simulink model "simple_wind_turbine_pmsg"  (Simulink 10.0)
settings: Solver=ode23tb  StartTime=0.0  StopTime=2  MaxStep=0.04  RelTol=1e-3  EnableMultiTasking=on
libraries: powerlib x5, simulink x1, powerlib_extras x1, re_lib x1
Description:
  | This model is developed to encourage the learner/student to develop a
  | Variable Speed Wind Turbine with PMSG. I considered basic parameters
  | in Matlab Blocks with little modification based on the output/load.
  | User can vary and simulate any parameter to study the response of
  | the system.
  | User can add a rectifier and a battery for battery storage system.
  | All the best.
  | mpaul.prasad@gmail.com
settings Model: Creator=PAUL SIR  LastModifiedBy=bhisma
settings DataIOCC: LimitDataPoints=on  SignalLoggingSaveFormat=ModelDataLogs
settings OptimizationCC: ExpressionDepthLimit=2147483647
settings DebuggingCC: SolverPrmCheckMsg=warning  FcnCallInpInsideContextMsg=warning  StateNameClashWarn=warning
settings GRTTargetCC: GeneratePreprocessorConditionals=Disable all  CombineOutputUpdateFcns=on  GRTInterface=off
settings ConfigComp: CovExternalEMLEnable=off
settings SimscapeCC: SimscapeNormalizeSystem=off

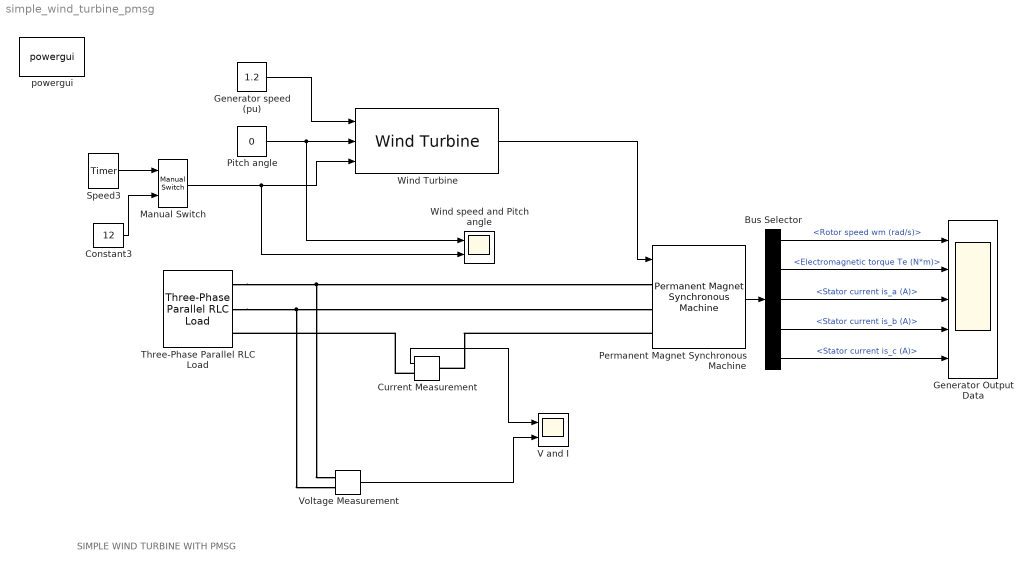
== system simple_wind_turbine_pmsg ==
  note: SIMPLE WIND TURBINE WITH PMSG
  Bus Selector : BusSelector  OutputSignals=Rotor speed wm (rad/s),Electromagnetic torque Te (N*m),Stator current is_a (A),Stator current is_b (A),Stator current is_c (A)
  Constant3 : Constant  Value=12
  Current Measurement : powerlib/Measurements/Current Measurement  PhasorSimulation=off  OutputType=Complex  PSBequivalent=0
      settings: SourceProductName=Simscape Electrical
  Generator Output Data : Scope  NumInputPorts=5
  Generator speed (pu) : Constant  Value=1.2
  Manual Switch : simulink/Signal Routing/Manual Switch  sw=0  action=0  varsize=off
      settings: SourceProductName=Simulink  SourceProductBaseCode=SL
  Permanent Magnet Synchronous Machine : powerlib/Machines/Permanent Magnet Synchronous Machine  NbPhases=3  FluxDistribution=Sinusoidal  RotorType=Round  MechanicalLoad=Torque Tm  PresetModel=No  ShowDetailedParameters=on  Resistance=0.0018  Inductance=8.5e-3  dqInductances=[8.5e-3,8.5e-3]  La=0.000835  MachineConstant=Voltage Constant (V_peak L-L / krpm)  Flux=0.55133  VoltageCst=400  TorqueCst=3.308  Flat=120  Mechanical=[0.00062 0.0003035 5 0]  PolePairs=5  InitialConditions=[0,0, 0,0]  InitialConditions5ph=[0 0 0 0 0 0]  TsPowergui=0  TsBlock=-1  RefAngle=90 degrees behind phase A axis (modified Park)
  Pitch angle : Constant  Value=0
  Speed3 : powerlib_extras/Control  Blocks/Timer  t=[0 1 2]  e=[12 8 12]
      settings: SourceProductName=Simscape Electrical  SourceProductBaseCode=PS
  Three-Phase Parallel RLC Load : powerlib/Elements/Three-Phase Parallel RLC Load  LConnTagsString=A|B|C  Configuration=Y (grounded)  NominalVoltage=400  NominalFrequency=50  ActivePower=110  InductivePower=0  CapacitivePower=0  Measurements=None  LoadType=constant Z
      settings: SourceProductName=Simscape Electrical
  V and I : Scope  NumInputPorts=2
  Voltage Measurement : powerlib/Measurements/Voltage Measurement  PhasorSimulation=off  OutputType=Complex  PSBequivalent=0
      settings: SourceProductName=Simscape Electrical
  Wind Turbine : re_lib/Wind Generation/Wind Turbine  Pnom=200  Pelec_base=200/0.9  wind_base=12  P_wind_base=0.73  speed_nom=1.2  pitch_angle=0  DisplayTurbChar=off  c1_c6="[0.51763          116          0.4            5           21     0.006795]"  cp_nom=0.48  lambda_nom=8.1
      settings: SourceProductName=Simscape Electrical  SourceProductBaseCode=PS
  Wind speed and Pitch angle : Scope  NumInputPorts=2
  powergui : powerlib/powergui  Priority=1  SimulationMode=Continuous  SolverType=Tustin  SampleTime=50e-6  frequency=60  SPID=off  DisableSnubberDevices=off  DisableRonSwitches=off  DisableVfSwitches=off  SwTol=0  Interpol=off  DisplayEquations=off  FunctionMessages=off  frequencyindice=0  Pbase=100e6  ErrMax=1e-4  Iterations=50  UnitsV=kV  UnitsW=MW  echomessages=off  HookPort=off  EnableUseOfTLC=off  x0status=blocks  RestoreLinks=warning  ResistiveCurrentMeasurement=off  Ylog=off  Xlog=on  ShowGrid=off  save=off  variable=ZData  ZoomFFT=off  StartTime=0.0  cycles=1  DisplayStyle=1  FreqAxis=off  MaxFrequency=1000  frequencyindicesteady=1  display=off  methode=off
      settings: SourceProductName=Simscape Electrical
  wires:
  Wind Turbine/1 -> Permanent Magnet Synchronous Machine/1
  Pitch angle/1 -> Wind Turbine/2, Wind speed and Pitch angle/1
  Generator speed (pu)/1 -> Wind Turbine/1
  Voltage Measurement/1 -> V and I/2
  Permanent Magnet Synchronous Machine/1 -> Bus Selector/1
  Bus Selector/1 -> Generator Output Data/1  "<Rotor speed wm (rad/s)>"
  Bus Selector/2 -> Generator Output Data/2  "<Electromagnetic torque Te (N*m)>"
  Bus Selector/3 -> Generator Output Data/3  "<Stator current is_a (A)>"
  Bus Selector/4 -> Generator Output Data/4  "<Stator current is_b (A)>"
  Bus Selector/5 -> Generator Output Data/5  "<Stator current is_c (A)>"
  Current Measurement/1 -> V and I/1
  Speed3/1 -> Manual Switch/1
  Constant3/1 -> Manual Switch/2
  Manual Switch/1 -> Wind Turbine/3, Wind speed and Pitch angle/2
  connections:
  Three-Phase Parallel RLC Load/LConn1 -- Permanent Magnet Synchronous Machine/LConn1 -- Voltage Measurement/LConn1
  Three-Phase Parallel RLC Load/LConn2 -- Permanent Magnet Synchronous Machine/LConn2 -- Voltage Measurement/LConn2
  Current Measurement/RConn1 -- Three-Phase Parallel RLC Load/LConn3
  Permanent Magnet Synchronous Machine/LConn3 -- Current Measurement/LConn1
